simulink model "YawController"  (R2026b)
settings: Solver=FixedStepDiscrete  StopTime=1.0  FixedStep=TorqueVectoringControlSampleTime
settings Model: DataDictionary=VehicleData.sldd  Creator=Xu Dingyi  LastModifiedBy=29358
settings DebuggingCC: AlgebraicLoopMsg=error

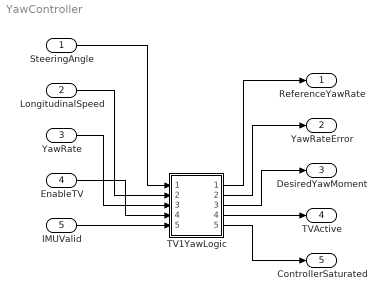
== system YawController ==
  SteeringAngle : Inport  OutDataTypeStr=double  Unit=rad
  LongitudinalSpeed : Inport  Port=2  OutDataTypeStr=double  Unit=m/s
  YawRate : Inport  Port=3  OutDataTypeStr=double  Unit=rad/s
  EnableTV : Inport  Port=4  OutDataTypeStr=boolean
  IMUValid : Inport  Port=5  OutDataTypeStr=boolean
  TV1YawLogic : Stateflow chart  TreatAsAtomicUnit=on
  ReferenceYawRate : Outport  OutDataTypeStr=double  Unit=rad/s
  YawRateError : Outport  Port=2  OutDataTypeStr=double  Unit=rad/s
  DesiredYawMoment : Outport  Port=3  OutDataTypeStr=double  Unit=N*m
  TVActive : Outport  Port=4  OutDataTypeStr=boolean
  ControllerSaturated : Outport  Port=5  OutDataTypeStr=boolean
  wires:
  SteeringAngle/1 -> TV1YawLogic/1(SteeringAngle)
  IMUValid/1 -> TV1YawLogic/5(IMUValid)
  EnableTV/1 -> TV1YawLogic/4(EnableTV)
  YawRate/1 -> TV1YawLogic/3(YawRate)
  LongitudinalSpeed/1 -> TV1YawLogic/2(LongitudinalSpeed)
  TV1YawLogic/1(ReferenceYawRate) -> ReferenceYawRate/1
  TV1YawLogic/3(DesiredYawMoment) -> DesiredYawMoment/1
  TV1YawLogic/2(YawRateError) -> YawRateError/1
  TV1YawLogic/4(TVActive) -> TVActive/1
  TV1YawLogic/5(ControllerSaturated) -> ControllerSaturated/1

== stateflow chart YawController/TV1YawLogic ==
  settings: updateMethod=DISCRETE  sampleTime=TorqueVectoringControlSampleTime
  state ActiveControl
    en: IntegratorState = 0;
    du: [ReferenceYawRate, YawRateError, DesiredYawMoment, TVActive, ControllerSaturated, IntegratorState] = torqueVectoringYawControlStep(SteeringAngle, LongitudinalSpeed, YawRate, EnableTV, IMUValid, IntegratorState, TorqueVectoringControlSampleTime, TorqueVectoringWheelbase, TorqueVectoringUndersteerGradient, TorqueVectoringMinimumControlSpeed, TorqueVectoringFrictionEstimate, TorqueVectoringGravity, TorqueVectoringLateralAccelerationLimit, TorqueVectoringYawRateLimit, TorqueVectoringYawKp, TorqueVectoringYawKi, TorqueVectoringYawAntiWindupGain, TorqueVectoringYawMomentLimit);
  (default) -> ActiveControl
  data: SteeringAngle input double; LongitudinalSpeed input double; YawRate input double; EnableTV input boolean; IMUValid input boolean; ReferenceYawRate output double; YawRateError output double; DesiredYawMoment output double; TVActive output boolean; ControllerSaturated output boolean; IntegratorState local double; TorqueVectoringControlSampleTime parameter double; TorqueVectoringWheelbase parameter double; TorqueVectoringUndersteerGradient parameter double; TorqueVectoringMinimumControlSpeed parameter double; TorqueVectoringFrictionEstimate parameter double; TorqueVectoringGravity parameter double; TorqueVectoringLateralAccelerationLimit parameter double; TorqueVectoringYawRateLimit parameter double; TorqueVectoringYawKp parameter double; TorqueVectoringYawKi parameter double; TorqueVectoringYawAntiWindupGain parameter double; TorqueVectoringYawMomentLimit parameter double
